simulink model "zy7gyz21"  (R2022a)
settings: Solver=VariableStepAuto  StartTime=0.0  StopTime=80  RelTol=1e-3
settings Model: Creator=dell  LastModifiedBy=dell

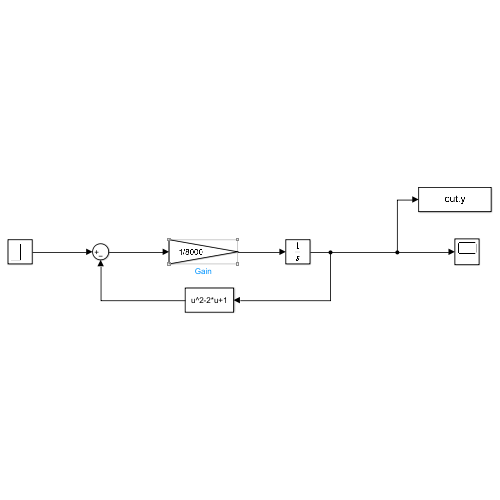
[thumbnail: Simulink's stored preview of the top-level diagram]
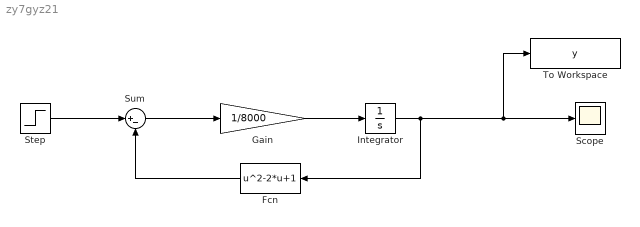
== system zy7gyz21 ==
  Fcn : Fcn  Expr=u^2-2*u+1
  Gain : Gain  Gain=1/8000
  Integrator : Integrator
  Scope : Scope
  Step : Step  Time=0  After=150000  SampleTime=0
  Sum : Sum  Inputs=|+-
  To Workspace : ToWorkspace  VariableName=y  SaveFormat=Timeseries  SampleTime=-1
  wires:
  Step/1 -> Sum/1
  Sum/1 -> Gain/1
  Gain/1 -> Integrator/1
  Integrator/1 -> Fcn/1, To Workspace/1, Scope/1
  Fcn/1 -> Sum/2
